simulink model "constraints_comparison_A_4D_v2_Fc_disconnected"  (R2017b)
settings: Solver=ode4  StartTime=0.0  StopTime=total_time  FixedStep=0.001  RelTol=1e-3  EnableMultiTasking=on
InitFcn:
  | % clear
  | % clc
  | 
  | wavelet_gen
undefined symbols (not defined in the file or in its folder): acm_aero_model, acm_T_N, breakpoints1, Cm0, Cmde, Cmq, comp_feedback, constraint_type, dail, de, dele, dele_trim, drud, FCdelay, firstimpulsewidth3211, firstimpulsewidthdoublet, Fr_mp_1, Fr_mp_2, Fr_rp_1, Fr_rp_2, ini_acm_de_deg, ini_acm_p_deg_per_s, ini_acm_phi_deg, ini_acm_psi_deg, ini_acm_q_deg_per_s, ini_acm_r_deg_per_s, ini_acm_theta_deg, ini_cmp_de_deg, ini_rig_p_deg_per_s, ini_rig_phi_deg, ini_rig_psi_deg, ini_rig_q_deg_per_s, ini_rig_r_deg_per_s, ini_rig_theta_deg, input_type, K1_svo_acm, K1_svo_cmp, K2_svo_acm, K2_svo_cmp, La, Ma, max_defl_sat_acm, max_defl_sat_cmp, max_rate_sat, max_rate_sat_acm, max_rate_sat_cmp, Na, radius, sigbuilder_block, simstop, theta_trim, thrust_trim, windspeed, Xa, Ya, Za
libraries: aerolibconvert2 x119, simulink x36, sharedtransform x19, vrlib x2
(part 5 of 6)

== matlab function constraints_comparison_A_4D_v2_Fc_disconnected/Subsystem14/Extracting position vector 3/MATLAB Function ==
  data: u input; y output
function y = fcn(u)
%#codegen

y = [   u(1)
        u(2)
        u(3)    ];

== matlab function constraints_comparison_A_4D_v2_Fc_disconnected/Subsystem14/MATLAB Function4 ==
  data: q2 output size=[4,1]; q1 input size=[7,1]
function q2  = fcn(q1)

q2 = q1(4:7,1);

== matlab function constraints_comparison_A_4D_v2_Fc_disconnected/Equations of motion ==
  data: qa input size=[7,1]; qa_dot_dot output size=[7,1]; qa_dot input size=[7,1]; cs_response input size=[3,1]; thrust input size=[1,1]; Fa output size=[3,1]; V output size=[1,1]; alpha output size=[1,1]; alpha_dot input size=[1,1]; beta output size=[1,1]; p output size=[1,1]; q output size=[1,1]; r output size=[1,1]; react output; F_c input size=[3,1]; radius output; param_states output; constraint_type input; comp_feedback input; radius input
function [qa_dot_dot, Fa, V,alpha,beta,p,q,r,react,radius,param_states] = fcn(qa, qa_dot,cs_response,thrust,alpha_dot,F_c,constraint_type,comp_feedback,radius)

%% Choose constraint type:
% 1 = unconstrained
% 2 = spherical constraint
% 3 = planar constraint
% 5 = position fixed

cons = constraint_type;

%% Compensator feedback
% 1 = on
% 0 = off

% comp_feedback = 1;

%% Constants
g = 9.81;

%% Control surfaces
dail = cs_response(1);
dele = cs_response(2);
drud = cs_response(3);

% %% Aircraft properties (Hawk)
% 
% m_a = 1.970; % 1.645; % kg
% Ixx_a = 0.008083; % 0.00959; % kg.m^2
% Iyy_a = 0.038; %0.047642; % 0.044; % kg.m^2
% Izz_a = 0.061206; % 0.0507; % kg.m^2
% Ixy_a = 0; % kg.m^2
% Ixz_a = 0; % kg.m^2
% Iyz_a = 0; % kg.m^2
% 
% % Position of body axes origin (c.g. position) relative to inertial axes origin in body frame of reference
% ua0 = [ 0.8*0
%         0.0
%         0.0  ];

%% Aircraft properties (A 4D, taken from Flight Stability and Automatic Control, Robert C. Nelson, 1989, page 254)

% Scale factor for subscale model (T. G. Gainer and S. Hoffman, Summary of Transformation Equations and Equations of Motion Used in Free-Flight and Wind-Tunnel Data Reduction and Analysis, NASA SP-3070, 1972)
m_a_hawk_rounded = 2.0; % kg
m_a_fullscale = 7973.2467;	% kg, 17578 lb
R_l = (m_a_hawk_rounded/m_a_fullscale)^(1/3); % (6.31% scale)
R_rho = 1; % Both aircraft are assumed to be at sea level

m_a = 7973.2467*R_rho*R_l^3;                % kg, 17578 lb              (6.31% scale: 2.0000 kg)
Ixx_a = 10968.5672*R_rho*R_l^5;             % kg.m^2, 8090 slug.ft^2    (6.31% scale: 0.0109 kg.m^2)
Iyy_a = 35115.6849*R_rho*R_l^5;             % kg.m^2, 25900 slug.ft^2   (6.31% scale: 0.0350 kg.m^2)
Izz_a = 39589.8841*R_rho*R_l^5;             % kg.m^2, 29200 slug.ft^2   (6.31% scale: 0.0395 kg.m^2)
Ixy_a = 0*R_rho*R_l^5;                      % kg.m^2                    (6.31% scale: 0.0000 kg.m^2)
Ixz_a = 1762.56333*R_rho*R_l^5;             % kg.m^2, 1300 slug.ft^2    (6.31% scale: 0.0018 kg.m^2)
Iyz_a = 0*R_rho*R_l^5;                      % kg.m^2                    (6.31% scale: 0.0000 kg.m^2)

% Position of body axes origin (c.g. position) relative to inertial axes origin in body frame of reference
ua0 = [ 0.8*0
        0.0
        0.0  ];
    
%% Input position and attitude vectors

Ra1 = qa(1);
Ra2 = qa(2);
Ra3 = qa(3);
qa0 = qa(4);
qa1 = qa(5);
qa2 = qa(6);
qa3 = qa(7);

%% Input linear and angular velocity vectors

Ra1_dot = qa_dot(1);
Ra2_dot = qa_dot(2);
Ra3_dot = qa_dot(3);
qa0_dot = qa_dot(4);
qa1_dot = qa_dot(5);
qa2_dot = qa_dot(6);
qa3_dot = qa_dot(7);

%% Transformation matrices
            
Ea = [  -qa1     qa0      -qa3     qa2
        -qa2     qa3      qa0      -qa1
        -qa3     -qa2     qa1      qa0  ];
    
E_dasha = [     -qa1     qa0      qa3      -qa2
                -qa2     -qa3     qa0      qa1
                -qa3     qa2      -qa1     qa0  ];
            
Aa = Ea*transpose(E_dasha);

%% Mass and inertial matrix (M) of system
        
% Mass matrix of aircraft model
Ma_RR = [   m_a	0   0
            0   m_a	0
            0   0   m_a	];
        
% Inertial tensor of aircraft model in body frame of reference about c.g./body axes
Ia = [   Ixx_a	-Ixy_a	-Ixz_a
        -Ixy_a	 Iyy_a	-Iyz_a
        -Ixz_a	-Iyz_a	 Izz_a	];
    
MMa = [  Ma_RR    	zeros(3,4)
        zeros(4,3)	transpose(2*E_dasha)*Ia*2*E_dasha	];
    
M = [   MMa  	];

%% Aerodynamics model

rho = 1.225;    % Density (kg/m^3)
% rho = 1.218;  % Density (kg/m^3) Bristol

% M = 0.4 at sea level (447 ft/sec (136.246 m/s, 6.31% scale: 34.2155 m/s), from Aircraft Stability and Control Data, Teper, 1969)
V_t = 30; % Tunnel windspeed (m/s)

%%% Calculating angle of attack (alpha), sideslip (sideslip) and local angular velocities (p, q, r)

% Velocity of aircraft in inertial axes
V_a_inertial = [    qa_dot(1)+V_t
                   	qa_dot(2)
                   	qa_dot(3)      ];
                    
V_a_inertial_pert = [  	qa_dot(1)
                      	qa_dot(2)
                       	qa_dot(3)      ];

% Velocity of aircraft in body axes (vector_inertial = A * vector_body, where A is the transformation matrix)
V_a_body = transpose(Aa)*V_a_inertial;
V_a_body_pert = transpose(Aa)*V_a_inertial_pert;

% Magnitude of total local velocity vector
V = sqrt((V_a_inertial(1))^2+(V_a_inertial(2))^2+(V_a_inertial(3))^2);

% Angle of attack (alpha)
alpha = atan2(V_a_body(3),V_a_body(1));

% Sideslip angle (beta)
beta = asin(V_a_body(2)/V);

% Local angular velocities (p, q, r in body axes)
omega_dasha = 2*E_dasha*[	qa0_dot
                            qa1_dot
                            qa2_dot
                            qa3_dot     ];
                        
p = omega_dasha(1);
q = omega_dasha(2);
r = omega_dasha(3);

% % Alpha_dot calculation
% u_body = V_a_body(1);
% w_body = V_a_body(3);
% u_dot_body = V_a_dot_body_pert(1);
% w_dot_body = V_a_dot_body_pert(3);
% alpha_dot = (w_dot_body*u_body - u_dot_body*w_body)/((u_body*sec(alpha))^2);
% % alpha_dot = (w_dot_body*u_body - u_dot_body*w_body)/(u_body^2 + w_body^2);

% Reference dimensions (Hawk)
c_hawk = 0.143;        % m
S_hawk = 0.084942;     % m^2
b_hawk = 0.594;        % m

% Reference dimensions (A 4D, taken from Flight Stability and Automatic Control, Robert C. Nelson, 1989, page 254)
c_a_fullscale = 3.29184;     	% m,    10.8 ft
S_a_fullscale = 24.1548;     	% m^2,  260 ft^2
b_a_fullscale = 8.382;          % m,    27.5 ft

% Scaled reference dimensions (to match mass of the Hawk, A 4D 6.31% scale)
c_a = c_a_fullscale*R_l;     	% m,    10.8 ft    	(0.2076 m)
S_a = S_a_fullscale*R_l^2;   	% m^2,  260 ft^2  	(0.0961 m^2)
b_a = b_a_fullscale*R_l;       	% m,    27.5 ft   	(0.5286 m)

% Longitudinal nondimensional derivatives (A 4D, M = 0.4, sea level, taken from Flight Stability and Automatic Control, Robert C. Nelson, 1989, page 254)
CL0             = 0.28;
CD0             = 0.03;
CL_alpha        = 3.45;
CD_alpha        = 0.30;
Cm_alpha        = -0.38;
CL_alpha_dot    = 0.72;
Cm_alpha_dot    = -1.1;
CL_q            = 0.0;
Cm_q            = -3.6;
CL_dele         = 0.36;
Cm_dele         = -0.50;

% Lateral dimensional derivatives (A 4D, M = 0.4, sea level, taken from Flight Stability and Automatic Control, Robert C. Nelson, 1989, page 254)
CY_beta         = -0.98;
Cl_beta         = -0.12;
Cn_beta         = 0.25;
Cl_p            = -0.26;
Cn_p            = 0.022;
Cl_r            = 0.14;
Cn_r            = -0.35;
Cl_dail         = -0.08;    % Sign changed for convention
Cn_dail         = -0.06;    % Sign changed for convention
CY_drud         = 0.17;
Cl_drud         = 0.105;    % Sign changed for convention
Cn_drud         = -0.032;  	% Sign changed for convention

CL = CL0 + CL_alpha*alpha + CL_alpha_dot*alpha_dot*(c_a/(2*V)) + CL_q*q*(c_a/(2*V)) + CL_dele*dele;
CD = CD0 + CD_alpha*alpha;
CY = CY_beta*beta + CY_drud*drud;
Cl = Cl_beta*beta + Cl_p*p*(b_a/(2*V)) + Cl_r*r*(b_a/(2*V)) + Cl_dail*dail + Cl_drud*drud;
Cm = Cm_alpha*alpha + Cm_alpha_dot*alpha_dot*(c_a/(2*V)) + Cm_q*q*(c_a/(2*V)) + Cm_dele*dele;
Cn = Cn_beta*beta + Cn_p*p*(b_a/(2*V)) + Cn_r*r*(b_a/(2*V)) + Cn_dail*dail + Cn_drud*drud;

% Body axis velocities (p, q, r are already defined above)
u = V_a_body_pert(1);
v = V_a_body_pert(2);
w = V_a_body_pert(3);
% w_dot = V_a_dot_dot_body_pert(3);

D_wind=0.5*rho*V^2*S_a*CD;
Y_wind=0.5*rho*V^2*S_a*CY;
L_wind=0.5*rho*V^2*S_a*CL;

l_wind=0.5*rho*V^2*S_a*b_a*Cl;
m_wind=0.5*rho*V^2*S_a*c_a*Cm;
n_wind=0.5*rho*V^2*S_a*b_a*Cn;

F_wind = [ -D_wind
            Y_wind
           -L_wind   ];
        
M_wind = [  l_wind
            m_wind
            n_wind   ];
        
% Body to wind axes transformation
% According to Cook (page 21): (phi,theta,psi) = (0,alpha,-beta)
phi_w = 0;
theta_w = alpha;
psi_w = -beta;

% From NASA transformation equations:
theta1 = psi_w;
theta2 = theta_w;
theta3 = phi_w;

q0 = +sin(theta1/2)*sin(theta2/2)*sin(theta3/2)+cos(theta1/2)*cos(theta2/2)*cos(theta3/2);
q1 = -sin(theta1/2)*sin(theta2/2)*cos(theta3/2)+sin(theta3/2)*cos(theta1/2)*cos(theta2/2);
q2 = +sin(theta1/2)*sin(theta3/2)*cos(theta2/2)+sin(theta2/2)*cos(theta1/2)*cos(theta3/2);
q3 = +sin(theta1/2)*cos(theta2/2)*cos(theta3/2)-sin(theta2/2)*sin(theta3/2)*cos(theta1/2);

E = [  -q1     q0      -q3     q2
        -q2     q3      q0      -q1
        -q3     -q2     q1      q0  ];
    
E_dash = [     -q1     q0      q3      -q2
                -q2     -q3     q0      q1
                -q3     q2      -q1     q0  ];
            
A_b2w = E*transpose(E_dash); % Note: this matrx transforms from body to wind axes!

% Body axes forces and moments
F_dash_a = transpose(A_b2w)*F_wind + [thrust;0;0];
M_dash_a = transpose(A_b2w)*M_wind;

% Inertial axes moments
F_a = Aa*F_dash_a;

%% Computing external forces matrix QE
                
% Angular velocity of aircraft model in body frame of reference
omega_dasha = 2*E_dasha*[	qa0_dot
                            qa1_dot
                            qa2_dot
                            qa3_dot     ];
                        
% External translational/linear forces on aircraft model in inertial frame of reference
% Fa1 = 0;
% Fa2 = 0;
% Fa3 = m_a*9.81;
Fa1 = F_a(1);
Fa2 = F_a(2);
Fa3 = F_a(3)+m_a*g;

switch comp_feedback
    case 1 % Compensator feedback force activated
        Fa = [  Fa1
                Fa2
                Fa3    ];

        Fa22 = Fa + F_c;
        
    otherwise % Compensator feedback force deactivated
        Fa = [  Fa1
                Fa2
                Fa3    ];

        Fa22 = Fa;
end

% External moments on aircraft model in body frame of reference
% Ma1 = 0;
% Ma2 = 0;
% Ma3 = 0;
Ma1 = M_dash_a(1);
Ma2 = M_dash_a(2);
Ma3 = M_dash_a(3);
Ma = [  Ma1
        Ma2
        Ma3     ];

QE_a = [    Fa22
            transpose(2*E_dasha)*(Ma-cross(omega_dasha,Ia*omega_dasha))	];
        
QE = [  QE_a    ];

%% Solving equations of motion

switch cons
        
    case 2 % Spherical constraint
        
        % Quaternion constriant
        Cq_1 = [	zeros(1,3)	qa0   qa1   qa2   qa3  ];
        QC_1 = -((qa0_dot)^2+(qa1_dot)^2+(qa2_dot)^2+(qa3_dot)^2);
        
        % Spherical constraint
        % radius = 0.8; % Sphere radius (m)
        Cq_2 = [    (Ra1+radius)   Ra2     Ra3     0   0   0   0];
        QC_2 = -Ra1_dot^2 - Ra2_dot^2 - Ra3_dot^2;
        
        Cq = [  Cq_1
                Cq_2  ];
        QC = [  QC_1
                QC_2  ];
        
    case 3 % Planar constraint
        
        % Quaternion constriant
        Cq_1 = [	zeros(1,3)	qa0   qa1   qa2   qa3  ];
        QC_1 = -((qa0_dot)^2+(qa1_dot)^2+(qa2_dot)^2+(qa3_dot)^2);
        
        % Planar constraint
        Cq_2 = [    1   0   0   0   0   0   0   ];
        QC_2 = 0;
        
        Cq = [  Cq_1
                Cq_2  ];
        QC = [  QC_1
                QC_2  ];
            
        radius = 0;
            
    case 4 % x and z constriant for validating lateral aerodynamics model
        
        % Quaternion constriant
        Cq_1 = [	zeros(1,3)	qa0   qa1   qa2   qa3  ];
        QC_1 = -((qa0_dot)^2+(qa1_dot)^2+(qa2_dot)^2+(qa3_dot)^2);
        
        % x constraint
        Cq_2 = [    1   0   0   0   0   0   0   ];
        QC_2 = 0;
        
     	% z constraint
        Cq_3 = [    0   0   1   0   0   0   0   ];
        QC_3 = 0;
        
        Cq = [  Cq_1
                Cq_2
                Cq_3  ];
        QC = [  QC_1
                QC_2
                QC_3  ];
            
        radius = 0;
            
	case 5 % x, y, z constriant (just to check)
        
        % Quaternion constriant
        Cq_1 = [	zeros(1,3)	qa0   qa1   qa2   qa3  ];
        QC_1 = -((qa0_dot)^2+(qa1_dot)^2+(qa2_dot)^2+(qa3_dot)^2);
        
        % x constraint
        Cq_2 = [    1   0   0   0   0   0   0   ];
        QC_2 = 0;
        
      	% y constraint
        Cq_3 = [    0   1   0   0   0   0   0   ];
        QC_3 = 0;
        
     	% z constraint
        Cq_4 = [    0   0   1   0   0   0   0   ];
        QC_4 = 0;
        
        Cq = [  Cq_1
                Cq_2
                Cq_3
                Cq_4	];
        QC = [  QC_1
                QC_2
                QC_3
                QC_4    ];
            
        radius = 0;
        
      	otherwise %case 1 % Unconstrained
        
        % Quaternion constriant
        Cq_1 = [	zeros(1,3)	qa0   qa1   qa2   qa3  ];
        QC_1 = -((qa0_dot)^2+(qa1_dot)^2+(qa2_dot)^2+(qa3_dot)^2);
        
        Cq = Cq_1;
        QC = QC_1;
        
        radius = 0;
        
end

        
MM = [  M   transpose(Cq)
        Cq  zeros(size(QC,1))        ];
QQ = [  QE
        QC  ];

qq = MM\QQ;

%% Output acceleration vectors
qa_dot_dot = qq(1:7);

%% Reaction loads
react = -transpose(Cq)*qq(end-size(Cq,1)+1:end);

%% States for parameter estimation

Ra1 = qa(1);
Ra2 = qa(2);
Ra3 = qa(3);
qa0 = qa(4);
qa1 = qa(5);
qa2 = qa(6);
qa3 = qa(7);

% From NASA transformation matrices (transformation 10)
% (vector_inertial = Aa * vector_body)
psi = atan2(Aa(2,1),Aa(1,1));
theta = atan2(-Aa(3,1),(sqrt(1-(Aa(3,1))^2)));
phi = atan2(Aa(3,2),Aa(3,3));

% Rotation rates in the body axes = [p, q, r]
rotation_rates_body = [p;q;r];
rotation_rates_inertial = Aa*rotation_rates_body;

% Rotation accelerations in the body axes = [p_dot, q_dot, r_dot]
rotation_acc_body = 2*E_dasha*qa_dot_dot(4:7);
% Another way of calculating body axes rotation rates and accelerations:
% q1 = qa(4:7);
% q_dot = qa_dot(4:7);
% q_dot_dot = qa_dot_dot(4:7);
% omega = 2*quatmultiply(q_dot',quatinv(q1'));
% omega_dot = 2*(quatmultiply(q_dot_dot',quatinv(q1')) - quatmultiply((0.5*omega),(0.5*omega)));
% rotation_acc_body = [omega_dot(2); omega_dot(3); omega_dot(4)];

param_states = [    qa(1) % x (m)
                    qa(2) % y (m)
                    qa(3) % z (m)
                    qa_dot(1) % x_dot (m/s)
                    qa_dot(2) % y_dot (m/s)
                    qa_dot(3) % z_dot (m/s)
                    qa_dot_dot(1) % x_dot_dot (m/s^2)
                    qa_dot_dot(2) % y_dot_dot (m/s^2)
                    qa_dot_dot(3) % z_dot_dot (m/s^2)
                    phi   % (rad)
                    theta % (rad)
                    psi   % (rad)
                    rotation_rates_body(1); % p (rad/sec)
                    rotation_rates_body(2); % q (rad/sec)
                    rotation_rates_body(3); % r (rad/sec)
                    rotation_acc_body(1); % p_dot (rad/sec^2)
                    rotation_acc_body(2); % q_dot (rad/sec^2)
                    rotation_acc_body(3); % r_dot (rad/sec^2)
                    m_a % Mass (kg)
                    Ixx_a % (kg.m^2)
                    Iyy_a % (kg.m^2)
                    Izz_a % (kg.m^2)
                    Ixy_a % (kg.m^2)
                    Ixz_a % (kg.m^2)
                    Iyz_a % (kg.m^2)
                    thrust % Thrust (N)
                    V_t % Freestream wind speed (m/s)
                    dail % Aileron (rad)
                    dele % Elevator (rad)
                   	drud % Rudder (rad)
                    b_a % Wing span (m)
                    c_a % Reference cord, MAC (m)
                    S_a % Wing area (m^2)
                    rho % Density (kg/m^3)
                    alpha_dot % (rad/s^2)
                    ];

== matlab function constraints_comparison_A_4D_v2_Fc_disconnected/Subsystem14/Subsystem13/MATLAB Function ==
  data: q input; x_ini output; y_ini output; z_ini output
function [x_ini,y_ini,z_ini]= fcn(q)

% Initial position

x = 0.8;
z = 0.1433;%0.03975;

p = [   x
        0
        z   ];

q0 = q(1);
q1 = q(2);
q2 = q(3);
q3 = q(4);

E = [  -q1     q0      -q3     q2
       -q2     q3      q0      -q1
       -q3     -q2     q1      q0  ];
    
E_dash = [     -q1     q0      q3      -q2
               -q2     -q3     q0      q1
               -q3     q2      -q1     q0  ];
           
A = E*transpose(E_dash);

p_in = A*p;

x_ini = p_in(1);
y_ini = p_in(2);
z_ini = p_in(3);

== matlab function constraints_comparison_A_4D_v2_Fc_disconnected/Subsystem14/Aircraft acceleration body axis ==
  data: Aa input; qa_dot_dot3 output; qa_dot_dot2 input; nz output
function [qa_dot_dot3,nz]= fcn(Aa, qa_dot_dot2)

% qa_dot_dot2 = linear accelerations in inertial frame
% qa_dot_dot3 = linear accelerations in body axis

qa_dot_dot3 = Aa\qa_dot_dot2;
% qa_dot_dot3 = qa_dot_dot2;

theta_acm = atan(-Aa(3,1)/sqrt(1-(Aa(3,1))^2));
nz = qa_dot_dot2(3)*cos(theta_acm)-qa_dot_dot2(1)*sin(theta_acm);

== matlab function constraints_comparison_A_4D_v2_Fc_disconnected/Subsystem14/Aerodynamics model: compensator ==
  data: qc input; V_t input; alpha input; beta input; q input; eta input; F_c output; M_dash_c output; r input; rudd input; extra output
function [F_c,M_dash_c,extra] = fcn(qc,V_t,alpha,beta,q,eta,r,rudd)

% beta = 0;

Rc1 = qc(1);
Rc2 = qc(2);
Rc3 = qc(3);
qc0 = qc(4);
qc1 = qc(5);
qc2 = qc(6);
qc3 = qc(7);

% Transformation matrices
Ec = [  -qc1     qc0      -qc3     qc2
        -qc2     qc3      qc0      -qc1
        -qc3     -qc2     qc1      qc0  ];
    
E_dashc = [     -qc1     qc0      qc3      -qc2
                -qc2     -qc3     qc0      qc1
                -qc3     qc2      -qc1     qc0  ];

Ac = Ec*transpose(E_dashc);

% Reference dimensions
c = 0.181;      % m
S = 0.1254;     % m^2
b = 0.7;        % m

% % Control surface deflection
% eta = dcs(1); % Virtual ailerons
% eta = dcs(2); % Virtual elevator
% eta = dcs(3); % Virtual rudder

% Aerodynamic coefficients (alpha = theta_rig)
% CL=3.647*alpha+1.306*eta+(2.302*0.181/V_t)*q; % Pattinson
% CL=2.18*alpha+0.5*eta+(b*15/(2*V_t))*q; % Matthew (old)
CL=1.73*alpha+1.42*eta+(b*4.69/(2*V_t))*q; % Matthew (13th Oct 2015)
% CD=CL^2/(3.907*pi); % Pattinson
CD=0; % Matthew
CM=0; % Pattinson/Matthew

% Side force
CY = 1.73*-beta+1.42*rudd+(b*4.69/(2*V_t))*r;

% Dynamic pressure
rho = 1.225;% 1.218; % Density (kg/m^3)
Dyn_p = 0.5*rho*V_t^2;

% Loads in wind axes (relative to total local velocity vector)
L = Dyn_p*S*CL;
D = Dyn_p*S*CD;
M = Dyn_p*S*c*CM;

Y = Dyn_p*S*CY;

% Transforming loads to body frame of reference from wind axes (See Cook p.21)
phi = 0;
theta = alpha;
psi = -beta;

% q0 = cos(phi/2)*cos(theta/2)*cos(psi/2)+sin(phi/2)*sin(theta/2)*sin(psi/2);
% q1 = cos(phi/2)*cos(theta/2)*sin(psi/2)-sin(phi/2)*sin(theta/2)*cos(psi/2);
% q2 = cos(phi/2)*sin(theta/2)*cos(psi/2)+sin(phi/2)*cos(theta/2)*sin(psi/2);
% q3 = sin(phi/2)*cos(theta/2)*cos(psi/2)-cos(phi/2)*sin(theta/2)*sin(psi/2);
% 
% E = [  -q1     q0      -q3     q2
%         -q2     q3      q0      -q1
%         -q3     -q2     q1      q0  ];
%     
% E_dash = [     -q1     q0      q3      -q2
%                 -q2     -q3     q0      q1
%                 -q3     q2      -q1     q0  ];
%             
% A = E*transpose(E_dash);

theta1 = psi;
theta2 = theta;
theta3 = phi;

q0 = +sin(theta1/2)*sin(theta2/2)*sin(theta3/2)+cos(theta1/2)*cos(theta2/2)*cos(theta3/2);
q1 = -sin(theta1/2)*sin(theta2/2)*cos(theta3/2)+sin(theta3/2)*cos(theta1/2)*cos(theta2/2);
q2 = +sin(theta1/2)*sin(theta3/2)*cos(theta2/2)+sin(theta2/2)*cos(theta1/2)*cos(theta3/2);
q3 = +sin(theta1/2)*cos(theta2/2)*cos(theta3/2)-sin(theta2/2)*sin(theta3/2)*cos(theta1/2);

E = [	-q1     q0      -q3     q2
        -q2     q3      q0      -q1
        -q3     -q2     q1      q0  ];
    
E_dash = [	-q1     q0      q3      -q2
           	-q2     -q3     q0      q1
           	-q3     q2      -q1     q0  ];
            
A10 = E*transpose(E_dash);
A10_transpose_inertial_to_body = A10';

F_dash_c = A10_transpose_inertial_to_body*[ -D
                                            Y
                                            -L  ];
                      
% M_dash_c = transpose(A)*[ 0
%                           M
%                           0   ];
M_dash_c = A10_transpose_inertial_to_body*[  0
                                             M
                                             0   ];
                    
% Transforming forces onto inertial frame
F_c = Ac*F_dash_c;

% F_c = [     -D*0
%             0
%             -L  ]; %/cos(alpha)

% F_c = zeros(3,1);
% M_dash_c = zeros(3,1);

%% Extra
extra = [   alpha*180/pi
            beta*180/pi
            -D
            Y
            -L
            F_dash_c
            F_c];

== matlab function constraints_comparison_A_4D_v2_Fc_disconnected/Subsystem14/MATLAB Function7 ==
  data: V_t output size=[1]; qc input size=[7,1]; theta_rig output size=[1]; p output; qc_dot input size=[7,1]; q output size=[1]; r output; qc_dot_dot input; Vt input; Vc output; omega_dashc_dot output
function [V_t,theta_rig,p,q,r,Vc,omega_dashc_dot] = fcn(qc,qc_dot,qc_dot_dot,Vt)
  
Rc1 = qc(1);
Rc2 = qc(2);
Rc3 = qc(3);
qc0 = qc(4);
qc1 = qc(5);
qc2 = qc(6);
qc3 = qc(7);

Rc1_dot = qc_dot(1);
Rc2_dot = qc_dot(2);
Rc3_dot = qc_dot(3);
qc0_dot = qc_dot(4);
qc1_dot = qc_dot(5);
qc2_dot = qc_dot(6);
qc3_dot = qc_dot(7);

Rc1_dot_dot = qc_dot_dot(1);
Rc2_dot_dot = qc_dot_dot(2);
Rc3_dot_dot = qc_dot_dot(3);
qc0_dot_dot = qc_dot_dot(4);
qc1_dot_dot = qc_dot_dot(5);
qc2_dot_dot = qc_dot_dot(6);
qc3_dot_dot = qc_dot_dot(7);

% Transformation matrices
Ec = [  -qc1     qc0      -qc3     qc2
        -qc2     qc3      qc0      -qc1
        -qc3     -qc2     qc1      qc0  ];
    
E_dashc = [     -qc1     qc0      qc3      -qc2
                -qc2     -qc3     qc0      qc1
                -qc3     qc2      -qc1     qc0  ];

Ac = Ec*transpose(E_dashc);

% Wind tunnel velocity vector
Vtt = [  Vt
         0   
         0   ];

% Velocity vector of aircraft model in inertial frame of reference
Vc = [  Rc1_dot
        Rc2_dot
        Rc3_dot	];

% Total velocity vector of aircraft model in body frame of reference
Vc_dash = transpose(Ac)*(Vc + Vtt);

% Magnitude of total local velocity vector
V0 = sqrt((Vc_dash(1))^2+(Vc_dash(2))^2+(Vc_dash(3))^2);

% Angle of attack
alpha = atan2(Vc_dash(3),Vc_dash(1));

% Acceleration in body frame
c_dash = transpose(Ac)*[    Rc1_dot_dot
                            Rc2_dot_dot
                            Rc3_dot_dot     ];

% Acceleration in z-direction body frame
w_dot = c_dash(3);

% Sideslip angle [CHECK SIGN]
beta = asin(Vc_dash(2)/V0);

% Local angular velocities
omega_dashc = 2*E_dashc*[	qc0_dot
                            qc1_dot
                            qc2_dot
                            qc3_dot     ];
                        
% Angular rate
p = omega_dashc(1); % rad/s
q = omega_dashc(2); % rad/s
r = omega_dashc(3); % rad/s

V_t = Vtt(1);

% Rig pitch angle
% theta_rig = atan2(-Ac(3,1),sqrt(1-(Ac(3,1))^2));
theta_rig = 0;

%% Local angular acceleration
omega_dashc_dot = 2*E_dashc*[	qc0_dot_dot
                            qc1_dot_dot
                            qc2_dot_dot
                            qc3_dot_dot     ];

== matlab function constraints_comparison_A_4D_v2_Fc_disconnected/Subsystem14/Aerodynamics model: Hawk ==
  data: Cm0 input; Cmde input; de input; Cmq input; T input; acm_aero_model input; qa input; V0 input; alpha input; w_dot input; q input; eta input; F_a output; M_dash_a output; q_rig input; Aa output
function [F_a,M_dash_a,Aa] = fcn(Cm0,Cmde,de,Cmq,T,acm_aero_model,qa,V0,alpha,w_dot,q,eta,q_rig)

beta = 0;

Ra1 = qa(1);
Ra2 = qa(2);
Ra3 = qa(3);
qa0 = qa(4);
qa1 = qa(5);
qa2 = qa(6);
qa3 = qa(7);

% Transformation matrices
Ea = [  -qa1     qa0      -qa3     qa2
        -qa2     qa3      qa0      -qa1
        -qa3     -qa2     qa1      qa0  ];
    
E_dasha = [     -qa1     qa0      qa3      -qa2
                -qa2     -qa3     qa0      qa1
                -qa3     qa2      -qa1     qa0  ];

Aa = Ea*transpose(E_dasha);

% Reference dimensions (Hawk)
c = 0.143;       % m
S = 0.084942;    % m^2

% theta_acm = atan(-Aa(3,1)/sqrt(1-(Aa(3,1))^2));
% aplha_approx = theta_acm -0.8*q_rig/30;

% Aerodynamic coefficients
% (Note: CL0=0.1155 is multiplied by a factor of 1.80 to match experimental
%  data)
% CL=0.1155*1.80/1.80+3.8004*alpha+0.4429*eta-0.4456*alpha*eta-4.447*alpha^2-0.04322*eta^2-7.314*alpha*eta^2-4.636*alpha^2*eta+0.0008039*alpha^3+0.001499*eta^3+1.828*q*c/V0*0+33*(c/(2*V0))*q+1.342*c/(V0^2)*w_dot*0;
% CD=0.04953+0.04801*alpha-0.008018*eta+0.4703*alpha*eta+1.669*alpha^2+0.3445*eta^2+0.2102*alpha*eta^2-0.9875*alpha^2*eta+0.00001016*alpha^3-0.00002714*eta^3;
% CM=0.04463-0.5919*alpha-0.7774*eta+0.4383*alpha*eta-0.1227*alpha^2-0.4214*eta^2-2.587*alpha*eta^2+3.292*alpha^2*eta-0.0001252*alpha^3-0.002631*eta^3-3.528*q*c/V0-2.604*c/(V0^2)*w_dot*0;

% CL=0.1155*0.75+3.8004*0.75*alpha+0.4429*0.75*eta-0.4456*alpha*eta-4.447*alpha^2-0.04322*eta^2-7.314*alpha*eta^2-4.636*alpha^2*eta+0.0008039*alpha^3+0.001499*eta^3-1.828*q*c/V0-1.342*c/(V0^2)*w_dot;
% CD=0.04953*0.75+0.04801*0.75*alpha-0.008018*0.75*eta+0.4703*alpha*eta+1.669*alpha^2+0.3445*eta^2+0.2102*alpha*eta^2-0.9875*alpha^2*eta+0.00001016*alpha^3-0.00002714*eta^3;
% CM=0.04463*0.75-0.5919*0.75*alpha-0.7774*0.75*eta+0.4383*alpha*eta-0.1227*alpha^2-0.4214*eta^2-2.587*alpha*eta^2+3.292*alpha^2*eta-0.0001252*alpha^3-0.002631*eta^3-3.528*q*c/V0-2.604*1/(V0^2)*w_dot

% CL = 0.1155*1.80 + 3.8*alpha + 0.4431009*eta + 33*(c/(2*V0))*q; % Linear model (Matthew)
% CD=0.04953+0.04801*alpha-0.008018*eta+0.4703*alpha*eta+1.669*alpha^2+0.3445*eta^2+0.2102*alpha*eta^2-0.9875*alpha^2*eta+0.00001016*alpha^3-0.00002714*eta^3;
% CD=0.04953+0.04801*alpha+1.669*alpha^2; % Simplified
% CM = Cm0 + Cmde*(eta-de) + Cmq*(c/(2*V0))*q; % Matthew's data (13th Oct 2015)

% V0 = 30;%%%%
% alpha2 = (theta_acm - 0.8*q_rig/30);%%%%

switch acm_aero_model
    case 1 % Nanjing
        CL=0.1155+3.8004*alpha+0.4429*eta-0.4456*alpha*eta-4.447*alpha^2-0.04322*eta^2-7.314*alpha*eta^2-4.636*alpha^2*eta+0.0008039*alpha^3+0.001499*eta^3-1.828*q*c/V0-1.342*c/(V0^2)*w_dot;
        CD=0.04953+0.04801*alpha-0.008018*eta+0.4703*alpha*eta+1.669*alpha^2+0.3445*eta^2+0.2102*alpha*eta^2-0.9875*alpha^2*eta+0.00001016*alpha^3-0.00002714*eta^3;
        CM=0.04463-0.5919*alpha-0.7774*eta+0.4383*alpha*eta-0.1227*alpha^2-0.4214*eta^2-2.587*alpha*eta^2+3.292*alpha^2*eta-0.0001252*alpha^3-0.002631*eta^3-3.528*q*c/V0-2.604*1/(V0^2)*w_dot;
    case 2 % Matthew's linear model
        CL = 0.1155*1.80 + 3.8*alpha + 0.4431009*eta + 33*(c/(2*V0))*q;
        CD = 0;
        CM = 0.04463 -0.528*alpha -8.14*(c/(2*V0))*q -0.84*eta;
    case 3 % Matthew's linear model + lookup table for CM
        CL = 0.1155*1.80 + 3.8*alpha + 0.4431009*eta + 33*(c/(2*V0))*q;
        CD = 0;
        CM = Cm0 + Cmde*(eta-de) + Cmq*(c/(2*V0))*q; % Matthew's data (13th Oct 2015)
    otherwise
        CL = 0;
        CD = 0;
        CM = 0;
end

% Dynamic pressure
rho = 1.225;%1.218; % Density (kg/m^3)
Dyn_p = 0.5*rho*V0^2;

% Loads in wind axes (relative to total local velocity vector)
L = Dyn_p*S*CL;
D = Dyn_p*S*CD;
M = Dyn_p*S*c*CM;

% Transforming loads to body frame of reference from wind axes (See Cook p.21, rotation sequence: 0->3 YAW, PITCH, ROLL)
phi = 0;
theta = alpha;
psi = -beta;

% q0 = cos(phi/2)*cos(theta/2)*cos(psi/2)+sin(phi/2)*sin(theta/2)*sin(psi/2);
% q1 = cos(phi/2)*cos(theta/2)*sin(psi/2)-sin(phi/2)*sin(theta/2)*cos(psi/2);
% q2 = cos(phi/2)*sin(theta/2)*cos(psi/2)+sin(phi/2)*cos(theta/2)*sin(psi/2);
% q3 = sin(phi/2)*cos(theta/2)*cos(psi/2)-cos(phi/2)*sin(theta/2)*sin(psi/2);

theta1 = psi;
theta2 = theta;
theta3 = phi;

q0 = +sin(theta1/2)*sin(theta2/2)*sin(theta3/2)+cos(theta1/2)*cos(theta2/2)*cos(theta3/2);
q1 = -sin(theta1/2)*sin(theta2/2)*cos(theta3/2)+sin(theta3/2)*cos(theta1/2)*cos(theta2/2);
q2 = +sin(theta1/2)*sin(theta3/2)*cos(theta2/2)+sin(theta2/2)*cos(theta1/2)*cos(theta3/2);
q3 = +sin(theta1/2)*cos(theta2/2)*cos(theta3/2)-sin(theta2/2)*sin(theta3/2)*cos(theta1/2);

E = [  -q1     q0      -q3     q2
        -q2     q3      q0      -q1
        -q3     -q2     q1      q0  ];
    
E_dash = [     -q1     q0      q3      -q2
                -q2     -q3     q0      q1
                -q3     q2      -q1     q0  ];
            
 A = E*transpose(E_dash); % body axes to inertial/wind axes transformation

% Free-flying model thrust (in body axes)
thrust = T; %3.55; %3.126;

F_dash_a2 = transpose(A)*[  -D
                            0
                            -L  ];
                      
F_dash_a = F_dash_a2 + [    thrust
                            0
                            0       ];
                    
M_dash_a = transpose(A)*[ 0
                          M
                          0   ];
                    
% Transforming forces onto inertial frame
F_a = Aa*F_dash_a;

% F_a = [ -D+thrust
%          0
%         -L  ]; % /cos(theta_acm)

% F_a = zeros(3,1);
% M_dash_a = zeros(3,1);

== matlab function constraints_comparison_A_4D_v2_Fc_disconnected/Subsystem14/MATLAB Function8 ==
  data: A3 input; A33 output
function A33 = fcn(A3)

A33 = [ A3(1,1)
        A3(2,1)
        A3(3,1)
        A3(1,2)
        A3(2,2)
        A3(3,2)
        A3(1,3)
        A3(2,3)
        A3(3,3) ];

== matlab function constraints_comparison_A_4D_v2_Fc_disconnected/Subsystem14/Aircraft_model_friction ==
  data: theta_dot_rp input; theta_dot_mp input; Fr_mp output; theta_dot_relative output
function [Fr_mp,theta_dot_relative] = fcn(theta_dot_rp,theta_dot_mp)

theta_dot_relative = theta_dot_mp-theta_dot_rp;

%% John Pattinson's friction model
% Fs_mp = 2.74E-4;
% Fc_mp = 1.68E-3;
% omega2_mp = 3.94E-4;
% 
% Fr_mp = [   0
%             -((sign(theta_dot)*(Fs_mp+Fc_mp)/2 + omega2_mp.*theta_dot))
%             0                                                                   ];
%         
% if abs(theta_dot) < 1E-3
%     Fr_mp = [   0
%             	0
%                 0	];
% end

%% Sergio's friction model (parameter estimation) 09-11-2015
% Model gimbal
k1m = 35.97e-3;
k2m = 0.239e-3;
k3m = 112e3;

Fr_mp = [   0
            -(k1m*theta_dot_relative + k2m*tanh(k3m*theta_dot_relative))
            0                                                                   ];

% if abs(theta_dot) < 1E-3
%     Fr_mp = [   0
%             	0
%                 0	];
% end

== matlab function constraints_comparison_A_4D_v2_Fc_disconnected/Subsystem14/Compensator friction ==
  data: theta_dot_rp input; Fr_rp output
function Fr_rp  = fcn(theta_dot_rp)

%% John Pattinson's friction model
% Fs_rp = 2.79E-2;
% Fc_rp = 3.39E-2;
% omega2_rp = 4.10E-3;
% 
% Fr_rp = [   0
%             -((sign(theta_dot_rp)*(Fs_rp+Fc_rp)/2 + omega2_rp.*theta_dot_rp))
%             0                                                                       ];

%% Sergio's friction model (parameter estimation) 09-11-2015
% Rig gimbal
k1r = 6.324e-3;
k2r = 24.42e-3;
k3r = 25;

Fr_rp = [   0
            -(k1r*theta_dot_rp + k2r*tanh(k3r*theta_dot_rp))
            0                                                                   ];

== matlab function constraints_comparison_A_4D_v2_Fc_disconnected/Subsystem14/Virtual compensator deflections to physical deflections ==
  data: da_cmp input; servo1 output; de_cmp input; dr_cmp input; servo2 output; servo3 output; servo4 output; s2 output; da_cmp2 output; de_cmp2 output; dr_cmp2 output
function [servo1,servo2,servo3,servo4,s2,da_cmp2,de_cmp2,dr_cmp2] = fcn(da_cmp, de_cmp, dr_cmp)

d = [   da_cmp
        de_cmp
        dr_cmp  ];
    
A = [   1    1  -1
        1   -1  -1
        1   -1   1
        1    1   1  ];
    
s = A*d;

servo1 = s(1);
servo2 = s(2);
servo3 = s(3);
servo4 = s(4);

% Limiting servo deflection
if servo1 > 40*pi/180
    servo1 = 40*pi/180;
end
if servo2 > 40*pi/180
    servo2 = 40*pi/180;
end
if servo3 > 40*pi/180
    servo3 = 40*pi/180;
end
if servo4 > 40*pi/180
    servo4 = 40*pi/180;
end

if servo1 < -40*pi/180
    servo1 = -40*pi/180;
end
if servo2 < -40*pi/180
    servo2 = -40*pi/180;
end
if servo3 < -40*pi/180
    servo3 = -40*pi/180;
end
if servo4 < -40*pi/180
    servo4 = -40*pi/180;
end

s2 = [ 	servo1
        servo2
        servo3
        servo4  ];
    
A = [   1    1  -1   1
        1   -1  -1  -1
        1   -1   1  +1
        1    1   1  -1  ];
    
% NOTE: last column on matrix A is redundant to make a square matrix for
% inversion
    
d = A\s2;

da_cmp2 = d(1); % Virtual ailerons not used because direct control surface defections are fed to roll model
de_cmp2 = d(2);
dr_cmp2 = d(3);

== matlab function constraints_comparison_A_4D_v2_Fc_disconnected/Subsystem14/Aircraft attitude relative to arm2 ==
  data: phi_acm output; theta_acm output; psi_acm output; phi_arm output; theta_arm output; psi_arm output; Ar input; Aa input; phi_relative output; qr input; qa input; theta_relative output; psi_relative output
function [phi_acm,theta_acm,psi_acm,phi_arm,theta_arm,psi_arm,phi_relative,theta_relative,psi_relative]= fcn(Ar, Aa, qr, qa)

% qa is the state vector of the aircraft model in the inertial frame
% So, qa in the aircraft model's body frame is:

% qa_b = Aa\qa(4:7,1);

% A = Aa/Ar; % [CORRECT]

% A = Ar/Aa; [WRONG]
A = transpose(Ar)*Aa; % [CORRECT]

% A = Ar*inv(Aa);


% Rotation sequence: yaw, pitch, roll [WRONG, DO NOT USE]
% phi_relative = atan(A(2,1)/A(1,1));
% theta_relative = atan(-A(3,1)/sqrt(1-(A(3,1))^2));
% psi_relative = atan(A(3,2)/A(3,3));

% Rotation sequence: roll, pitch, yaw [CORRECT, SEE 'Rotation_sequence_check.m']
% phi_relative = atan(-A(2,3)/A(3,3));
% theta_relative = atan(A(1,3)/sqrt(1-(A(1,3))^2));
% psi_relative = atan(-A(1,2)/A(1,1));

% phi_acm = atan(-Aa(2,3)/Aa(3,3));
% theta_acm = atan(Aa(1,3)/sqrt(1-(Aa(1,3))^2));
% psi_acm = atan(-Aa(1,2)/Aa(1,1));
% 
% phi_arm = atan(-Ar(2,3)/Ar(3,3));
% theta_arm = atan(Ar(1,3)/sqrt(1-(Ar(1,3))^2));
% psi_arm = atan(-Ar(1,2)/Ar(1,1));

% The rotation sequence of the model-arm gimbal is actually: yaw, pitch, roll
% psi_relative = atan(A(2,1)/A(1,1));
% theta_relative = atan(-A(3,1)/sqrt(1-(A(3,1))^2));
% phi_relative = atan(A(3,2)/A(3,3));
% 
% psi_acm = atan(Aa(2,1)/Aa(1,1));
% theta_acm = atan(-Aa(3,1)/sqrt(1-(Aa(3,1))^2));
% phi_acm = atan(Aa(3,2)/A(3,3));
% 
% psi_arm = atan(Ar(2,1)/Ar(1,1));
% theta_arm = atan(-Ar(3,1)/sqrt(1-(Ar(3,1))^2));
% phi_arm = atan(Ar(3,2)/Ar(3,3));
psi_relative = atan2(A(2,1),A(1,1));
theta_relative = atan2(-A(3,1),sqrt(1-(A(3,1))^2));
phi_relative = atan2(A(3,2),A(3,3));

psi_acm = atan2(Aa(2,1),Aa(1,1));
theta_acm = atan2(-Aa(3,1),sqrt(1-(Aa(3,1))^2));
phi_acm = atan2(Aa(3,2),A(3,3));

psi_arm = atan2(Ar(2,1),Ar(1,1));
theta_arm = atan2(-Ar(3,1),sqrt(1-(Ar(3,1))^2));
phi_arm = atan2(Ar(3,2),Ar(3,3));

== matlab function constraints_comparison_A_4D_v2_Fc_disconnected/Subsystem14/Physical deflections to virtual compensator deflections ==
  data: da_cmp output; servo1 input; de_cmp output; dr_cmp output; servo2 input; servo3 input; servo4 input
function [da_cmp, de_cmp, dr_cmp] = fcn(servo1,servo2,servo3,servo4)

s = [   servo1
        servo2
        servo3
        servo4  ];
    
A = [   1    1  -1   1
        1   -1  -1  -1
        1   -1   1  +1
        1    1   1  -1  ];
    
% NOTE: last column on matrix A is redundant to make a square matrix for
% inversion
    
d = A\s;

da_cmp = d(1);
de_cmp = d(2);
dr_cmp = d(3);

== matlab function constraints_comparison_A_4D_v2_Fc_disconnected/Integrator for velocity/MATLAB Function ==
  data: p_rig input; u_ini output; v_ini output; w_ini output; q_rig input; r_rig input; q1 input; qr input; p_acm input; q_dot output; q_acm input; r_acm input
function [u_ini,v_ini,w_ini,q_dot]= fcn(p_rig,q_rig,r_rig,q1,qr,p_acm,q_acm,r_acm)

% Initial position

% r = 0.8;
% 
% x_ini = r*cos(theta_rig);
% y_ini = 0;
% z_ini = -r*sin(theta_rig);
% 
% u_ini = q_rig*z_ini; 
% v_ini = 0;
% w_ini = -q_rig*x_ini;

% Initial position
x_ini = 0.95*0;
y_ini = 0;
z_ini = 0;

% Local velocities in body axes (Cook, pg.74)
u_ini_body = q_rig*z_ini - r_rig*y_ini;
v_ini_body = r_rig*x_ini - p_rig*z_ini;
w_ini_body = p_rig*y_ini - q_rig*x_ini;

q00 = qr(4);
q11 = qr(5);
q22 = qr(6);
q33 = qr(7);

E = [  -q11     q00      -q33     q22
        -q22     q33      q00      -q11
        -q33     -q22     q11      q00  ];
    
E_dash = [     -q11     q00      q33      -q22
                -q22     -q33     q00      q11
                -q33     q22      -q11     q00  ];

% Body to inertial axes
A = E*transpose(E_dash);

% Inertial axes velocity
V_inertial = A*[    u_ini_body  
                    v_ini_body  
                    w_ini_body      ];
                
u_ini = V_inertial(1);
v_ini = V_inertial(2);
w_ini = V_inertial(3);

q = [   q1(4)
        q1(5)
        q1(6)
        q1(7)    ];

Q = [   -q(2)   -q(3)   -q(4)
        q(1)    -q(4)   q(3)
        q(4)    q(1)    -q(2)
        -q(3)   q(2)    q(1)    ];

omega = [   p_acm
            q_acm
            r_acm       ];

q_dot = 0.5*Q*omega;

== matlab function constraints_comparison_A_4D_v2_Fc_disconnected/Integrator for position/MATLAB Function ==
  data: q input; x_ini output; y_ini output; z_ini output
function [x_ini,y_ini,z_ini]= fcn(q)

% Initial position

r = 0.8*0;

p = [   r
        0
        0   ];

q0 = q(1);
q1 = q(2);
q2 = q(3);
q3 = q(4);

E = [  -q1     q0      -q3     q2
       -q2     q3      q0      -q1
       -q3     -q2     q1      q0  ];
    
E_dash = [     -q1     q0      q3      -q2
               -q2     -q3     q0      q1
               -q3     q2      -q1     q0  ];
           
A = E*transpose(E_dash);

p_in = A*p;

x_ini = p_in(1);
y_ini = p_in(2);
z_ini = p_in(3);

== matlab function constraints_comparison_A_4D_v2_Fc_disconnected/Extracting position vector 3/MATLAB Function ==
  data: u input; y output
function y = fcn(u)
%#codegen

y = [   u(1)
        u(2)
        u(3)    ];

== matlab function constraints_comparison_A_4D_v2_Fc_disconnected/Extracting position vector 3/MATLAB Function6 ==
  data: A3 input; A33 output
function A33 = fcn(A3)

A33 = [ A3(1,1)
        A3(2,1)
        A3(3,1)
        A3(1,2)
        A3(2,2)
        A3(3,2)
        A3(1,3)
        A3(2,3)
        A3(3,3) ];

== matlab function constraints_comparison_A_4D_v2_Fc_disconnected/Extracting position vector 3/MATLAB Function1 ==
  data: qa input; Aa output
function Aa = fcn(qa)
%% Input position and attitude vectors
qa0 = qa(4);
qa1 = qa(5);
qa2 = qa(6);
qa3 = qa(7);

%% Transformation matrices
            
Ea = [  -qa1     qa0      -qa3     qa2
        -qa2     qa3      qa0      -qa1
        -qa3     -qa2     qa1      qa0  ];
    
E_dasha = [     -qa1     qa0      qa3      -qa2
                -qa2     -qa3     qa0      qa1
                -qa3     qa2      -qa1     qa0  ];
            
Aa = Ea*transpose(E_dasha);

== matlab function constraints_comparison_A_4D_v2_Fc_disconnected/Subsystem14/Subsystem10/MATLAB Function ==
  data: p_rig input; u_ini output; v_ini output; w_ini output; q_rig input; r_rig input; q1 input; q_dot output
function [u_ini,v_ini,w_ini,q_dot]= fcn(p_rig,q_rig,r_rig, q1)

% Initial position

% x = 0.8;
% z = 0.3183;
% 
% theta_pos = atan(z/x) - theta_rig;
% r = sqrt(x^2+z^2);
% 
% u_ini = q_rig*r*sin(theta_pos); 
% v_ini = 0;
% w_ini = -q_rig*r*cos(theta_pos);
% 
% q = [   q1(4)
%         q1(5)
%         q1(6)
%         q1(7)    ];
% 
% Q = [   -q(2)   -q(3)   -q(4)
%         q(1)    -q(4)   q(3)
%         q(4)    q(1)    -q(2)
%         -q(3)   q(2)    q(1)    ];
% 
% omega = [   0
%             q_rig
%             0       ];
% 
% q_dot = 0.5*Q*omega;

% Initial position
x_ini = 0.95;
y_ini = 0;
z_ini = 0.3183;

% Local velocities in body axes (Cook, pg.74)
u_ini_body = q_rig*z_ini - r_rig*y_ini;
v_ini_body = r_rig*x_ini - p_rig*z_ini;
w_ini_body = p_rig*y_ini - q_rig*x_ini;

q00 = q1(4);
q11 = q1(5);
q22 = q1(6);
q33 = q1(7);

E = [  -q11     q00      -q33     q22
        -q22     q33      q00      -q11
        -q33     -q22     q11      q00  ];
    
E_dash = [     -q11     q00      q33      -q22
                -q22     -q33     q00      q11
                -q33     q22      -q11     q00  ];

% Body to inertial axes
A = E*transpose(E_dash);

% Inertial axes velocity
V_inertial = A*[    u_ini_body  
                    v_ini_body  
                    w_ini_body      ];
                
u_ini = V_inertial(1);
v_ini = V_inertial(2);
w_ini = V_inertial(3);

q = [   q1(4)
        q1(5)
        q1(6)
        q1(7)    ];

Q = [   -q(2)   -q(3)   -q(4)
        q(1)    -q(4)   q(3)
        q(4)    q(1)    -q(2)
        -q(3)   q(2)    q(1)    ];

omega = [   p_rig
            q_rig
            r_rig       ];

q_dot = 0.5*Q*omega;

== matlab function constraints_comparison_A_4D_v2_Fc_disconnected/Calculating Yin and Zin using acceleration, and Xin using radial reaction force ==
  data: X_in output; qa_dot_dot input size=[7,1]; qa_dot input size=[7,1]; Y_in output size=[1,1]; Z_in output size=[1,1]; qa input size=[7,1]; radial_reaction input; F_c output; r input; X_in_rad output; cos_theta2 output; pos output
function [X_in,Y_in,Z_in,F_c,X_in_rad,cos_theta2,pos] = fcn(qa_dot_dot,qa_dot,qa,radial_reaction,r)

%% Calculating Y_in and Z_in (inertial axes) using tangential acceleration and aircraft position of the sphere
% Note: This assumes that the tangential component of X_in is cancelled by F_c

% Aircraft accelerations in inertial axes (m/s^2)
u_dot = qa_dot_dot(1);
v_dot = qa_dot_dot(2);
w_dot = qa_dot_dot(3);
acc = [u_dot; v_dot; w_dot];

% WARNING: Make sure the aircraft acceleration is the same as measured with the IMU, does it include centripetal acceleration?

% Aircraft velocity in inertial axes (m/s)
u = qa_dot(1);
v = qa_dot(2);
w = qa_dot(3);
vel = [u; v; w];

% Aircraft position on the sphere (m)
x = qa(1);
y = qa(2);
z = qa(3);
% r = 0.8; % Sphere radius (m)
pos = [x+r; y; z];

% "Rig" angular velocity (lin_vel = ang_vel*r)
lin_vel = norm(vel); % Linear acceleration magnitude
ang_vel = lin_vel/r; % Angular acceleration magnitude

% Centripetal acceleration vector (positive radially outward)
cen_acc = -r*ang_vel^2*pos./norm(pos);

% Tangential acceleration (because the total acceleration has a component in the radial direction due to the centripetal acceleration)
tan_acc = acc - cen_acc;

% Unit vector for the direction of tangential acceleration
dir_acc = tan_acc/norm(tan_acc);

% "Rig" angular acceleration (tan_acc = ang_acc*r)
ang_acc = norm(tan_acc)/r; % Angular acceleration magnitude

% Magnitude of tanjential force acting on aircraft (Moment = inertia * angular acceleration)
m = 2.0; % Mass of aircraft model (kg)
lin_F = m*r*ang_acc; % Linear force (N), this force acts in the same direction as the angular acceleration (ang_acc)

% Using dot product to find the components of the force acting in the Y and Z inertial directions
vec_F = lin_F*dir_acc; % Tangential force vector
perp1 = cross(pos,vec_F); % Orthogonal vector to tangential force and position
perp2 = cross(perp1,[1; 0; 0]); % Orthogonal vector to perp1 and inertial X direction [1; 0; 0], i.e. vector on the Y,Z plane
F = lin_F/(dot(perp2/norm(perp2),dir_acc)) * perp2/norm(perp2); % Force on Y,Z plane
Y_dir = [0; 1; 0]; % Y direction inertial (unit vector)
Z_dir = [0; 0; 1]; % Z direction inertial (unit vector)
Y_in = dot(F,Y_dir); % Tangential force resolved into the Y direction
Z_in = dot(F,Z_dir); % Tangential force resolved into the Z direction

% WARNING: If X_in is created by the aircraft, theta can reach 90 deg cause Y_in and Z_in to infinity!

% Check to make sure acceleration vector and position vector (on the sphere) is perpendicular
check = dot(tan_acc,pos); % This should be zero

%% Calculating F_c using the previously calculated Y_in and Z_in

% Total radial reaction force = centripetal - X_in_rad - Y_in_rad - Z_in_rad
% Therefore, X_in_rad = -(Total radial reaction force + Y_in_rad + Z_in_rad - centripetal)
rad_react = dot(radial_reaction,pos/norm(pos)); % Scalar radial reaction force measured by the load cell (postive radially outward)
X_in_rad = -dot((rad_react*pos/norm(pos) + dot((Y_in*Y_dir+Z_in*Z_dir),pos/norm(pos))*pos/norm(pos) - m*cen_acc),pos/norm(pos));

X_dir = [1; 0; 0]; % X direction inertial (unit vector)

cos_theta = dot(X_dir,pos/norm(pos));
cos_theta2 = (dot(perp2/norm(perp2),dir_acc));

% X_in becomes infinity (singularity) because dot(X_dir,pos/norm(pos)) goes to zero when theta = 90 deg (cos(90)=0)
X_in = X_in_rad/(dot(X_dir,pos/norm(pos))); % X_in magnitude (scalar) in the inertial axes

% if dot(X_dir,pos/norm(pos)) < 0.1
%     X_in = 0;
% else
%     X_in = X_in_rad/(dot(X_dir,pos/norm(pos))); % X_in magnitude (scalar) in the inertial axes
% end
% if X_in_rad < 0.1 && X_in_rad > -0.1
%     X_in = 0;
% else
%     X_in = X_in_rad/(dot(X_dir,pos/norm(pos))); % X_in magnitude (scalar) in the inertial axes
% end

X_in_tan = X_in*X_dir - X_in_rad*pos/norm(pos); % Tangential component of X_in
F_c = -X_in_tan; % Compensator force to cancel out X_in_tan
check = dot(F_c,pos); % Tangent check, should be zero

== matlab function constraints_comparison_A_4D_v2_Fc_disconnected/Calculating radial reaction force measured from load cell ==
  data: qa_dot input size=[7,1]; qa input size=[7,1]; F_ext input size=[3,1]; radial_reaction1 output; react input; radial_reaction2 output; r input
function [radial_reaction1,radial_reaction2] = fcn(qa_dot,qa,F_ext,react,r)

%% Calculating the radial reaction force measured by the load cell

% Aircraft velocity in inertial axes (m/s)
u = qa_dot(1);
v = qa_dot(2);
w = qa_dot(3);
vel = [u; v; w];

% Aircraft position on the sphere (m)
x = qa(1);
y = qa(2);
z = qa(3);
% r = 0.8; % Sphere radius (m)
pos = [x+r; y; z];

% "Rig" angular velocity (lin_vel = ang_vel*r)
lin_vel = norm(vel); % Linear acceleration magnitude
ang_vel = lin_vel/r; % Angular acceleration magnitude

% Centripetal force vector (positive radially outward)
cen_acc = -r*ang_vel^2*pos./norm(pos); % Centripetal velocity
m = 2.0; % Mass of aircraft model (kg)
cen_F = m*cen_acc; % Centripetal force vector

% Radial component of the aircraft external forces (acting radially outward)
F_rad = dot(F_ext,pos./norm(pos))*pos./norm(pos);

% Total radial reaction force measured using the load cell (positive radially outward)
radial_reaction1 = cen_F - F_rad; % Radial reaction force, calculated
radial_reaction2 = dot(react(1:3),pos./norm(pos))*pos./norm(pos); % Radial reacton force, from simulation (same as calculated!)

== matlab function constraints_comparison_A_4D_v2_Fc_disconnected/norm ==
  data: u input; y output
function y = fcn(u)

y = norm(u);

== matlab function constraints_comparison_A_4D_v2_Fc_disconnected/Subsystem14/Subsystem1/MATLAB Function ==
  data: q input; x_ini output; y_ini output; z_ini output
function [x_ini,y_ini,z_ini]= fcn(q)

% Initial position

r = -0.38-0.3*0;

p = [   r
        0
        0   ];

q0 = q(1);
q1 = q(2);
q2 = q(3);
q3 = q(4);

E = [  -q1     q0      -q3     q2
       -q2     q3      q0      -q1
       -q3     -q2     q1      q0  ];
    
E_dash = [     -q1     q0      q3      -q2
               -q2     -q3     q0      q1
               -q3     q2      -q1     q0  ];
           
A = E*transpose(E_dash);

p_in = A*p;

x_ini = p_in(1);
y_ini = p_in(2);
z_ini = p_in(3);

== matlab function constraints_comparison_A_4D_v2_Fc_disconnected/Subsystem14/Subsystem3/MATLAB Function ==
  data: q input; x_ini output; y_ini output; z_ini output
function [x_ini,y_ini,z_ini]= fcn(q)

% Initial position

x = 0.129; % 0.169;  % 0.2615;
z = 0.178; % 0.219;  % 0.109;

p = [   x
        0
        z   ];

q0 = q(1);
q1 = q(2);
q2 = q(3);
q3 = q(4);

E = [  -q1     q0      -q3     q2
       -q2     q3      q0      -q1
       -q3     -q2     q1      q0  ];
    
E_dash = [     -q1     q0      q3      -q2
               -q2     -q3     q0      q1
               -q3     q2      -q1     q0  ];
           
A = E*transpose(E_dash);

p_in = A*p;

x_ini = p_in(1);
y_ini = p_in(2);
z_ini = p_in(3);
